simulink model "c00007M_harness"  (R2018a)
settings: Solver=FixedStepAuto  StartTime=0.0  StopTime=300  FixedStep=0.1  RelTol=1e-3
undefined symbols (not defined in the file): A1, hmax, R1, R2, sigbuilder_block, TempThreshold
(part 1 of 14)
settings Model: Creator=aarrieta  LastModifiedBy=umarkiegi

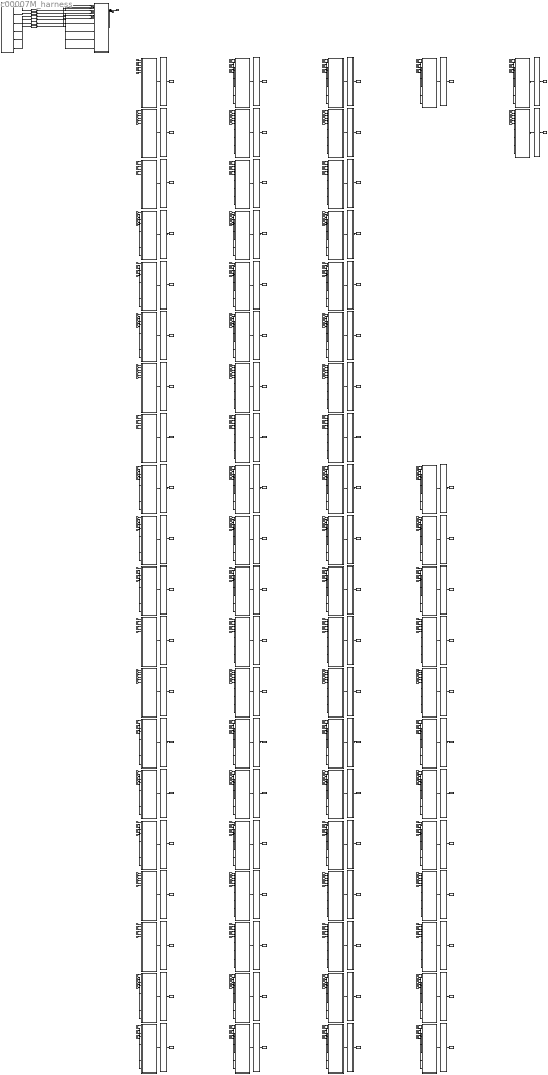
== system c00007M_harness ==
  CPSUT : Subsystem
  Eval : Subsystem
  Eval1 : Subsystem
  Eval10 : Subsystem
  Eval11 : Subsystem
  Eval12 : Subsystem
  Eval13 : Subsystem
  Eval14 : Subsystem
  Eval15 : Subsystem
  Eval16 : Subsystem
  Eval17 : Subsystem
  Eval18 : Subsystem
  Eval19 : Subsystem
  Eval2 : Subsystem
  Eval20 : Subsystem
  Eval21 : Subsystem
  Eval22 : Subsystem
  Eval23 : Subsystem
  Eval24 : Subsystem
  Eval25 : Subsystem
  Eval26 : Subsystem
  Eval27 : Subsystem
  Eval28 : Subsystem
  Eval29 : Subsystem
  Eval3 : Subsystem
  Eval30 : Subsystem
  Eval31 : Subsystem
  Eval32 : Subsystem
  Eval33 : Subsystem
  Eval34 : Subsystem
  Eval35 : Subsystem
  Eval36 : Subsystem
  Eval37 : Subsystem
  Eval38 : Subsystem
  Eval39 : Subsystem
  Eval4 : Subsystem
  Eval40 : Subsystem
  Eval41 : Subsystem
  Eval42 : Subsystem
  Eval43 : Subsystem
  Eval44 : Subsystem
  Eval45 : Subsystem
  Eval46 : Subsystem
  Eval47 : Subsystem
  Eval48 : Subsystem
  Eval49 : Subsystem
  Eval5 : Subsystem
  Eval50 : Subsystem
  Eval51 : Subsystem
  Eval52 : Subsystem
  Eval53 : Subsystem
  Eval54 : Subsystem
  Eval55 : Subsystem
  Eval56 : Subsystem
  Eval57 : Subsystem
  Eval58 : Subsystem
  Eval59 : Subsystem
  Eval6 : Subsystem
  Eval60 : Subsystem
  Eval68 : Subsystem
  Eval69 : Subsystem
  Eval7 : Subsystem
  Eval70 : Subsystem
  Eval71 : Subsystem
  Eval72 : Subsystem
  Eval73 : Subsystem
  Eval74 : Subsystem
  Eval75 : Subsystem
  Eval76 : Subsystem
  Eval77 : Subsystem
  Eval78 : Subsystem
  Eval79 : Subsystem
  Eval8 : Subsystem
  Eval80 : Subsystem
  Eval81 : Subsystem
  Eval9 : Subsystem
  Inputs : Subsystem  Tag=STV Subsys  LoadFcn=sigbuilder_block('load');  StartFcn=sigbuilder_block('start');  StopFcn=sigbuilder_block('stop');  ClipboardFcn=sigbuilder_block('clipboard');  mask(Sigbuilder block){tuvar=[0:10]}
      mask init:
      | if ~strcmp(get_param(bdroot(gcb),'SimulationStatus'),'stopped'),tuvar = sigbuilder_block('maskInit'); end
      settings: CopyFcn=sigbuilder_block('copy');  DeleteFcn=sigbuilder_block('delete');  ModelCloseFcn=sigbuilder_block('modelClose');  PreSaveFcn=sigbuilder_block('preSave');  PauseFcn=sigbuilder_block('pause');  ContinueFcn=sigbuilder_block('continue');  NameChangeFcn=sigbuilder_block('namechange');  OpenFcn=sigbuilder_block('open',[276.75 163.5 675.75 486.75 ]);  CloseFcn=sigbuilder_block('close');
      mask Display: plot(0, 0, 100, 100,[2, 2, 32, 32, 2], [68, 8, 8, 68, 68],[32, 2], [38, 38], [32, 19, 2],[53, 60, 44], [32, 17, 17, 2],[16, 16, 31, 31]);txt = getActiveGroup(gcbh);text(2, 100, txt,'verticalAlignment', 'top');
  M001 : Subsystem
  M002 : Subsystem
  M003 : Subsystem
  M004 : Subsystem
  M005 : Subsystem
  M006 : Subsystem
  M007 : Subsystem
  M008 : Subsystem
  M009 : Subsystem
  M010 : Subsystem
  M011 : Subsystem
  M012 : Subsystem
  M013 : Subsystem
  M014 : Subsystem
  M015 : Subsystem
  M016 : Subsystem
  M017 : Subsystem
  M018 : Subsystem
  M019 : Subsystem
  M020 : Subsystem
  M021 : Subsystem
  M022 : Subsystem
  M023 : Subsystem
  M024 : Subsystem
  M025 : Subsystem
  M026 : Subsystem
  M027 : Subsystem
  M028 : Subsystem
  M029 : Subsystem
  M030 : Subsystem
  M031 : Subsystem
  M032 : Subsystem
  M033 : Subsystem
  M034 : Subsystem
  M035 : Subsystem
  M036 : Subsystem
  M037 : Subsystem
  M038 : Subsystem
  M039 : Subsystem
  M040 : Subsystem
  M041 : Subsystem
  M042 : Subsystem
  M043 : Subsystem
  M044 : Subsystem
  M045 : Subsystem
  M046 : Subsystem
  M047 : Subsystem
  M048 : Subsystem
  M049 : Subsystem
  M050 : Subsystem
  M051 : Subsystem
  M052 : Subsystem
  M053 : Subsystem
  M054 : Subsystem
  M055 : Subsystem
  M056 : Subsystem
  M057 : Subsystem
  M058 : Subsystem
  M059 : Subsystem
  M060 : Subsystem
  M061 : Subsystem
  M069 : Subsystem
  M070 : Subsystem
  M071 : Subsystem
  M072 : Subsystem
  M073 : Subsystem
  M074 : Subsystem
  M075 : Subsystem
  M076 : Subsystem
  M077 : Subsystem
  M078 : Subsystem
  M079 : Subsystem
  M080 : Subsystem
  M081 : Subsystem
  M082 : Subsystem
  To Workspace : ToWorkspace  VariableName=mutant001  SampleTime=-1
  To Workspace1 : ToWorkspace  VariableName=mutant002  SampleTime=-1
  To Workspace10 : ToWorkspace  VariableName=mutant011  SampleTime=-1
  To Workspace11 : ToWorkspace  VariableName=mutant012  SampleTime=-1
  To Workspace12 : ToWorkspace  VariableName=mutant013  SampleTime=-1
  To Workspace13 : ToWorkspace  VariableName=mutant014  SampleTime=-1
  To Workspace14 : ToWorkspace  VariableName=mutant015  SampleTime=-1
  To Workspace15 : ToWorkspace  VariableName=mutant016  SampleTime=-1
  To Workspace16 : ToWorkspace  VariableName=mutant017  SampleTime=-1
  To Workspace17 : ToWorkspace  VariableName=mutant018  SampleTime=-1
  To Workspace18 : ToWorkspace  VariableName=mutant019  SampleTime=-1
  To Workspace19 : ToWorkspace  VariableName=mutant020  SampleTime=-1
  To Workspace2 : ToWorkspace  VariableName=mutant003  SampleTime=-1
  To Workspace20 : ToWorkspace  VariableName=mutant021  SampleTime=-1
  To Workspace21 : ToWorkspace  VariableName=mutant022  SampleTime=-1
  To Workspace22 : ToWorkspace  VariableName=mutant023  SampleTime=-1
  To Workspace23 : ToWorkspace  VariableName=mutant024  SampleTime=-1
  To Workspace24 : ToWorkspace  VariableName=mutant025  SampleTime=-1
  To Workspace25 : ToWorkspace  VariableName=mutant026  SampleTime=-1
  To Workspace26 : ToWorkspace  VariableName=mutant027  SampleTime=-1
  To Workspace27 : ToWorkspace  VariableName=mutant028  SampleTime=-1
  To Workspace28 : ToWorkspace  VariableName=mutant029  SampleTime=-1
  To Workspace29 : ToWorkspace  VariableName=mutant030  SampleTime=-1
  To Workspace3 : ToWorkspace  VariableName=mutant004  SampleTime=-1
  To Workspace30 : ToWorkspace  VariableName=mutant031  SampleTime=-1
  To Workspace31 : ToWorkspace  VariableName=mutant032  SampleTime=-1
  To Workspace32 : ToWorkspace  VariableName=mutant033  SampleTime=-1
  To Workspace33 : ToWorkspace  VariableName=mutant034  SampleTime=-1
  To Workspace34 : ToWorkspace  VariableName=mutant035  SampleTime=-1
  To Workspace35 : ToWorkspace  VariableName=mutant036  SampleTime=-1
  To Workspace36 : ToWorkspace  VariableName=mutant037  SampleTime=-1
  To Workspace37 : ToWorkspace  VariableName=mutant038  SampleTime=-1
  To Workspace38 : ToWorkspace  VariableName=mutant039  SampleTime=-1
  To Workspace39 : ToWorkspace  VariableName=mutant040  SampleTime=-1
  To Workspace4 : ToWorkspace  VariableName=mutant005  SampleTime=-1
  To Workspace40 : ToWorkspace  VariableName=mutant041  SampleTime=-1
  To Workspace41 : ToWorkspace  VariableName=mutant042  SampleTime=-1
  To Workspace42 : ToWorkspace  VariableName=mutant043  SampleTime=-1
  To Workspace43 : ToWorkspace  VariableName=mutant044  SampleTime=-1
  To Workspace44 : ToWorkspace  VariableName=mutant045  SampleTime=-1
  To Workspace45 : ToWorkspace  VariableName=mutant046  SampleTime=-1
  To Workspace46 : ToWorkspace  VariableName=mutant047  SampleTime=-1
  To Workspace47 : ToWorkspace  VariableName=mutant048  SampleTime=-1
  To Workspace48 : ToWorkspace  VariableName=mutant049  SampleTime=-1
  To Workspace49 : ToWorkspace  VariableName=mutant050  SampleTime=-1
  To Workspace5 : ToWorkspace  VariableName=mutant006  SampleTime=-1
  To Workspace50 : ToWorkspace  VariableName=mutant051  SampleTime=-1
  To Workspace51 : ToWorkspace  VariableName=mutant052  SampleTime=-1
  To Workspace52 : ToWorkspace  VariableName=mutant053  SampleTime=-1
  To Workspace53 : ToWorkspace  VariableName=mutant054  SampleTime=-1
  To Workspace54 : ToWorkspace  VariableName=mutant055  SampleTime=-1
  To Workspace55 : ToWorkspace  VariableName=mutant056  SampleTime=-1
  To Workspace56 : ToWorkspace  VariableName=mutant057  SampleTime=-1
  To Workspace57 : ToWorkspace  VariableName=mutant058  SampleTime=-1
  To Workspace58 : ToWorkspace  VariableName=mutant059  SampleTime=-1
  To Workspace59 : ToWorkspace  VariableName=mutant060  SampleTime=-1
  To Workspace6 : ToWorkspace  VariableName=mutant007  SampleTime=-1
  To Workspace60 : ToWorkspace  VariableName=mutant061  SampleTime=-1
  To Workspace68 : ToWorkspace  VariableName=mutant069  SampleTime=-1
  To Workspace69 : ToWorkspace  VariableName=mutant070  SampleTime=-1
  To Workspace7 : ToWorkspace  VariableName=mutant008  SampleTime=-1
  To Workspace70 : ToWorkspace  VariableName=mutant071  SampleTime=-1
  To Workspace71 : ToWorkspace  VariableName=mutant072  SampleTime=-1
  To Workspace72 : ToWorkspace  VariableName=mutant073  SampleTime=-1
  To Workspace73 : ToWorkspace  VariableName=mutant074  SampleTime=-1
  To Workspace74 : ToWorkspace  VariableName=mutant075  SampleTime=-1
  To Workspace75 : ToWorkspace  VariableName=mutant076  SampleTime=-1
  To Workspace76 : ToWorkspace  VariableName=mutant077  SampleTime=-1
  To Workspace77 : ToWorkspace  VariableName=mutant078  SampleTime=-1
  To Workspace78 : ToWorkspace  VariableName=mutant079  SampleTime=-1
  To Workspace79 : ToWorkspace  VariableName=mutant080  SampleTime=-1
  To Workspace8 : ToWorkspace  VariableName=mutant009  SampleTime=-1
  To Workspace80 : ToWorkspace  VariableName=mutant081  SampleTime=-1
  To Workspace81 : ToWorkspace  VariableName=mutant082  SampleTime=-1
  To Workspace9 : ToWorkspace  VariableName=mutant010  SampleTime=-1
  dtc_CT1 : DataTypeConversion
  dtc_E1 : DataTypeConversion
  dtc_EB1 : DataTypeConversion
  dtc_F1 : DataTypeConversion
  dtc_MR1 : DataTypeConversion
  dtc_T1 : DataTypeConversion
  LL1 : Outport
  tag scope: out1=global
  wires:
  CPSUT/1(LL1) -> [out1], LL1/1
  [in1] -> M001/1(CT1)
  [in2] -> M001/2(F1)
  [in3] -> M001/3(E1)
  [in4] -> M001/4(MR1)
  [in5] -> M001/5(T1)
  [in6] -> M001/6(EB1)
  Eval/1(Out1) -> To Workspace/1
  M001/1(LL1) -> Eval/1(In1)
  [in1] -> M002/1(CT1)
  [in2] -> M002/2(F1)
  [in3] -> M002/3(E1)
  [in4] -> M002/4(MR1)
  [in5] -> M002/5(T1)
  [in6] -> M002/6(EB1)
  M002/1(LL1) -> Eval1/1(In1)
  Eval1/1(Out1) -> To Workspace1/1
  [in1] -> M003/1(CT1)
  [in2] -> M003/2(F1)
  [in3] -> M003/3(E1)
  [in4] -> M003/4(MR1)
  [in5] -> M003/5(T1)
  [in6] -> M003/6(EB1)
  M003/1(LL1) -> Eval2/1(In1)
  Eval2/1(Out1) -> To Workspace2/1
  [in1] -> M004/1(CT1)
  [in2] -> M004/2(F1)
  [in3] -> M004/3(E1)
  [in4] -> M004/4(MR1)
  [in5] -> M004/5(T1)
  [in6] -> M004/6(EB1)
  M004/1(LL1) -> Eval3/1(In1)
  Eval3/1(Out1) -> To Workspace3/1
  [in1] -> M005/1(CT1)
  [in2] -> M005/2(F1)
  [in3] -> M005/3(E1)
  [in4] -> M005/4(MR1)
  [in5] -> M005/5(T1)
  [in6] -> M005/6(EB1)
  M005/1(LL1) -> Eval4/1(In1)
  Eval4/1(Out1) -> To Workspace4/1
  [in1] -> M006/1(CT1)
  [in2] -> M006/2(F1)
  [in3] -> M006/3(E1)
  [in4] -> M006/4(MR1)
  [in5] -> M006/5(T1)
  [in6] -> M006/6(EB1)
  M006/1(LL1) -> Eval5/1(In1)
  Eval5/1(Out1) -> To Workspace5/1
  [in1] -> M007/1(CT1)
  [in2] -> M007/2(F1)
  [in3] -> M007/3(E1)
  [in4] -> M007/4(MR1)
  [in5] -> M007/5(T1)
  [in6] -> M007/6(EB1)
  M007/1(LL1) -> Eval6/1(In1)
  Eval6/1(Out1) -> To Workspace6/1
  [in1] -> M008/1(CT1)
  [in2] -> M008/2(F1)
  [in3] -> M008/3(E1)
  [in4] -> M008/4(MR1)
  [in5] -> M008/5(T1)
  [in6] -> M008/6(EB1)
  M008/1(LL1) -> Eval7/1(In1)
  Eval7/1(Out1) -> To Workspace7/1
  [in1] -> M009/1(CT1)
  [in2] -> M009/2(F1)
  [in3] -> M009/3(E1)
  [in4] -> M009/4(MR1)
  [in5] -> M009/5(T1)
  [in6] -> M009/6(EB1)
  M009/1(LL1) -> Eval8/1(In1)
  Eval8/1(Out1) -> To Workspace8/1
  [in1] -> M010/1(CT1)
  [in2] -> M010/2(F1)
  [in3] -> M010/3(E1)
  [in4] -> M010/4(MR1)
  [in5] -> M010/5(T1)
  [in6] -> M010/6(EB1)
  M010/1(LL1) -> Eval9/1(In1)
  Eval9/1(Out1) -> To Workspace9/1
  [in1] -> M011/1(CT1)
  [in2] -> M011/2(F1)
  [in3] -> M011/3(E1)
  [in4] -> M011/4(MR1)
  [in5] -> M011/5(T1)
  [in6] -> M011/6(EB1)
  M011/1(LL1) -> Eval10/1(In1)
  Eval10/1(Out1) -> To Workspace10/1
  [in1] -> M012/1(CT1)
  [in2] -> M012/2(F1)
  [in3] -> M012/3(E1)
  [in4] -> M012/4(MR1)
  [in5] -> M012/5(T1)
  [in6] -> M012/6(EB1)
  M012/1(LL1) -> Eval11/1(In1)
  Eval11/1(Out1) -> To Workspace11/1
  [in1] -> M013/1(CT1)
  [in2] -> M013/2(F1)
  [in3] -> M013/3(E1)
  [in4] -> M013/4(MR1)
  [in5] -> M013/5(T1)
  [in6] -> M013/6(EB1)
  M013/1(LL1) -> Eval12/1(In1)
  Eval12/1(Out1) -> To Workspace12/1
  [in1] -> M014/1(CT1)
  [in2] -> M014/2(F1)
  [in3] -> M014/3(E1)
  [in4] -> M014/4(MR1)
  [in5] -> M014/5(T1)
  [in6] -> M014/6(EB1)
  M014/1(LL1) -> Eval13/1(In1)
  Eval13/1(Out1) -> To Workspace13/1
  [in1] -> M015/1(CT1)
  [in2] -> M015/2(F1)
  [in3] -> M015/3(E1)
  [in4] -> M015/4(MR1)
  [in5] -> M015/5(T1)
  [in6] -> M015/6(EB1)
  M015/1(LL1) -> Eval14/1(In1)
  Eval14/1(Out1) -> To Workspace14/1
  [in1] -> M016/1(CT1)
  [in2] -> M016/2(F1)
  [in3] -> M016/3(E1)
  [in4] -> M016/4(MR1)
  [in5] -> M016/5(T1)
  [in6] -> M016/6(EB1)
  M016/1(LL1) -> Eval15/1(In1)
  Eval15/1(Out1) -> To Workspace15/1
  [in1] -> M017/1(CT1)
  [in2] -> M017/2(F1)
  [in3] -> M017/3(E1)
  [in4] -> M017/4(MR1)
  [in5] -> M017/5(T1)
  [in6] -> M017/6(EB1)
  M017/1(LL1) -> Eval16/1(In1)
  Eval16/1(Out1) -> To Workspace16/1
  [in1] -> M018/1(CT1)
  [in2] -> M018/2(F1)
  [in3] -> M018/3(E1)
  [in4] -> M018/4(MR1)
  [in5] -> M018/5(T1)
  [in6] -> M018/6(EB1)
  M018/1(LL1) -> Eval17/1(In1)
  Eval17/1(Out1) -> To Workspace17/1
  [in1] -> M019/1(CT1)
  [in2] -> M019/2(F1)
  [in3] -> M019/3(E1)
  [in4] -> M019/4(MR1)
  [in5] -> M019/5(T1)
  [in6] -> M019/6(EB1)
  M019/1(LL1) -> Eval18/1(In1)
  Eval18/1(Out1) -> To Workspace18/1
  [in1] -> M020/1(CT1)
  [in2] -> M020/2(F1)
  [in3] -> M020/3(E1)
  [in4] -> M020/4(MR1)
  [in5] -> M020/5(T1)
  [in6] -> M020/6(EB1)
  M020/1(LL1) -> Eval19/1(In1)
  Eval19/1(Out1) -> To Workspace19/1
  [in1] -> M021/1(CT1)
  [in2] -> M021/2(F1)
  [in3] -> M021/3(E1)
  [in4] -> M021/4(MR1)
  [in5] -> M021/5(T1)
  [in6] -> M021/6(EB1)
  M021/1(LL1) -> Eval20/1(In1)
  Eval20/1(Out1) -> To Workspace20/1
  [in1] -> M022/1(CT1)
  [in2] -> M022/2(F1)
  [in3] -> M022/3(E1)
  [in4] -> M022/4(MR1)
  [in5] -> M022/5(T1)
  [in6] -> M022/6(EB1)
  M022/1(LL1) -> Eval21/1(In1)
  Eval21/1(Out1) -> To Workspace21/1
  [in1] -> M023/1(CT1)
  [in2] -> M023/2(F1)
  [in3] -> M023/3(E1)
  [in4] -> M023/4(MR1)
  [in5] -> M023/5(T1)
  [in6] -> M023/6(EB1)
  M023/1(LL1) -> Eval22/1(In1)
  Eval22/1(Out1) -> To Workspace22/1
  [in1] -> M024/1(CT1)
  [in2] -> M024/2(F1)
  [in3] -> M024/3(E1)
  [in4] -> M024/4(MR1)
  [in5] -> M024/5(T1)
  [in6] -> M024/6(EB1)
  M024/1(LL1) -> Eval23/1(In1)
  Eval23/1(Out1) -> To Workspace23/1
  [in1] -> M025/1(CT1)
  [in2] -> M025/2(F1)
  [in3] -> M025/3(E1)
  [in4] -> M025/4(MR1)
  [in5] -> M025/5(T1)
  [in6] -> M025/6(EB1)
  M025/1(LL1) -> Eval24/1(In1)
  Eval24/1(Out1) -> To Workspace24/1
  [in1] -> M026/1(CT1)
  [in2] -> M026/2(F1)
  [in3] -> M026/3(E1)
  [in4] -> M026/4(MR1)
  [in5] -> M026/5(T1)
  [in6] -> M026/6(EB1)
  M026/1(LL1) -> Eval25/1(In1)
  Eval25/1(Out1) -> To Workspace25/1
  [in1] -> M027/1(CT1)
  [in2] -> M027/2(F1)
  [in3] -> M027/3(E1)
  [in4] -> M027/4(MR1)
  [in5] -> M027/5(T1)
  [in6] -> M027/6(EB1)
  M027/1(LL1) -> Eval26/1(In1)
  Eval26/1(Out1) -> To Workspace26/1
  [in1] -> M028/1(CT1)
  [in2] -> M028/2(F1)
  [in3] -> M028/3(E1)
  [in4] -> M028/4(MR1)
  [in5] -> M028/5(T1)
  [in6] -> M028/6(EB1)
  M028/1(LL1) -> Eval27/1(In1)
  Eval27/1(Out1) -> To Workspace27/1
  [in1] -> M029/1(CT1)
  [in2] -> M029/2(F1)
  [in3] -> M029/3(E1)
  [in4] -> M029/4(MR1)
  [in5] -> M029/5(T1)
  [in6] -> M029/6(EB1)
  M029/1(LL1) -> Eval28/1(In1)
  Eval28/1(Out1) -> To Workspace28/1
  [in1] -> M030/1(CT1)
  [in2] -> M030/2(F1)
  [in3] -> M030/3(E1)
  [in4] -> M030/4(MR1)
  [in5] -> M030/5(T1)
  [in6] -> M030/6(EB1)
  M030/1(LL1) -> Eval29/1(In1)
  Eval29/1(Out1) -> To Workspace29/1
  [in1] -> M031/1(CT1)
  [in2] -> M031/2(F1)
  [in3] -> M031/3(E1)
  [in4] -> M031/4(MR1)
  [in5] -> M031/5(T1)
  [in6] -> M031/6(EB1)
  M031/1(LL1) -> Eval30/1(In1)
  Eval30/1(Out1) -> To Workspace30/1
  [in1] -> M032/1(CT1)
  [in2] -> M032/2(F1)
  [in3] -> M032/3(E1)
  [in4] -> M032/4(MR1)
  [in5] -> M032/5(T1)
  [in6] -> M032/6(EB1)
  M032/1(LL1) -> Eval31/1(In1)
  Eval31/1(Out1) -> To Workspace31/1
  [in1] -> M033/1(CT1)
  [in2] -> M033/2(F1)
  [in3] -> M033/3(E1)
  [in4] -> M033/4(MR1)
  [in5] -> M033/5(T1)
  [in6] -> M033/6(EB1)
  M033/1(LL1) -> Eval32/1(In1)
  Eval32/1(Out1) -> To Workspace32/1
  [in1] -> M034/1(CT1)
  [in2] -> M034/2(F1)
  [in3] -> M034/3(E1)
  [in4] -> M034/4(MR1)
  [in5] -> M034/5(T1)
  [in6] -> M034/6(EB1)
  M034/1(LL1) -> Eval33/1(In1)
  Eval33/1(Out1) -> To Workspace33/1
  [in1] -> M035/1(CT1)
  [in2] -> M035/2(F1)
  [in3] -> M035/3(E1)
  [in4] -> M035/4(MR1)
  [in5] -> M035/5(T1)
  [in6] -> M035/6(EB1)
  M035/1(LL1) -> Eval34/1(In1)
  Eval34/1(Out1) -> To Workspace34/1
  [in1] -> M036/1(CT1)
  [in2] -> M036/2(F1)
  [in3] -> M036/3(E1)
  [in4] -> M036/4(MR1)
  [in5] -> M036/5(T1)
  [in6] -> M036/6(EB1)
  M036/1(LL1) -> Eval35/1(In1)
  Eval35/1(Out1) -> To Workspace35/1
  [in1] -> M037/1(CT1)
  [in2] -> M037/2(F1)
  [in3] -> M037/3(E1)
  [in4] -> M037/4(MR1)
  [in5] -> M037/5(T1)
  [in6] -> M037/6(EB1)
  M037/1(LL1) -> Eval36/1(In1)
  Eval36/1(Out1) -> To Workspace36/1
  [in1] -> M038/1(CT1)
  [in2] -> M038/2(F1)
  [in3] -> M038/3(E1)
  [in4] -> M038/4(MR1)
  [in5] -> M038/5(T1)
  [in6] -> M038/6(EB1)
  M038/1(LL1) -> Eval37/1(In1)
  Eval37/1(Out1) -> To Workspace37/1
  [in1] -> M039/1(CT1)
  [in2] -> M039/2(F1)
  [in3] -> M039/3(E1)
  [in4] -> M039/4(MR1)
  [in5] -> M039/5(T1)
  [in6] -> M039/6(EB1)
  M039/1(LL1) -> Eval38/1(In1)
  Eval38/1(Out1) -> To Workspace38/1
  [in1] -> M040/1(CT1)
  [in2] -> M040/2(F1)
  [in3] -> M040/3(E1)
  [in4] -> M040/4(MR1)
  [in5] -> M040/5(T1)
  [in6] -> M040/6(EB1)
  M040/1(LL1) -> Eval39/1(In1)
  Eval39/1(Out1) -> To Workspace39/1
  [in1] -> M041/1(CT1)
  [in2] -> M041/2(F1)
  [in3] -> M041/3(E1)
  [in4] -> M041/4(MR1)
  [in5] -> M041/5(T1)
  [in6] -> M041/6(EB1)
  M041/1(LL1) -> Eval40/1(In1)
  Eval40/1(Out1) -> To Workspace40/1
  [in1] -> M042/1(CT1)
  [in2] -> M042/2(F1)
  [in3] -> M042/3(E1)
  [in4] -> M042/4(MR1)
  [in5] -> M042/5(T1)
  [in6] -> M042/6(EB1)
  M042/1(LL1) -> Eval41/1(In1)
  Eval41/1(Out1) -> To Workspace41/1
  [in1] -> M043/1(CT1)
  [in2] -> M043/2(F1)
  [in3] -> M043/3(E1)
  [in4] -> M043/4(MR1)
  [in5] -> M043/5(T1)
  [in6] -> M043/6(EB1)
  M043/1(LL1) -> Eval42/1(In1)
  Eval42/1(Out1) -> To Workspace42/1
  [in1] -> M044/1(CT1)
  [in2] -> M044/2(F1)
  [in3] -> M044/3(E1)
  [in4] -> M044/4(MR1)
  [in5] -> M044/5(T1)
  [in6] -> M044/6(EB1)
  M044/1(LL1) -> Eval43/1(In1)
  Eval43/1(Out1) -> To Workspace43/1
  [in1] -> M045/1(CT1)
  [in2] -> M045/2(F1)
  [in3] -> M045/3(E1)
  [in4] -> M045/4(MR1)
  [in5] -> M045/5(T1)
  [in6] -> M045/6(EB1)
  M045/1(LL1) -> Eval44/1(In1)
  Eval44/1(Out1) -> To Workspace44/1
  [in1] -> M046/1(CT1)
  [in2] -> M046/2(F1)
  [in3] -> M046/3(E1)
  [in4] -> M046/4(MR1)
  [in5] -> M046/5(T1)
  [in6] -> M046/6(EB1)
  M046/1(LL1) -> Eval45/1(In1)
  Eval45/1(Out1) -> To Workspace45/1
  [in1] -> M047/1(CT1)
  [in2] -> M047/2(F1)
  [in3] -> M047/3(E1)
  [in4] -> M047/4(MR1)
  [in5] -> M047/5(T1)
  [in6] -> M047/6(EB1)
  M047/1(LL1) -> Eval46/1(In1)
  Eval46/1(Out1) -> To Workspace46/1
  [in1] -> M048/1(CT1)
  [in2] -> M048/2(F1)
  [in3] -> M048/3(E1)
  [in4] -> M048/4(MR1)
  [in5] -> M048/5(T1)
  [in6] -> M048/6(EB1)
  M048/1(LL1) -> Eval47/1(In1)
  Eval47/1(Out1) -> To Workspace47/1
  [in1] -> M049/1(CT1)
  [in2] -> M049/2(F1)
  [in3] -> M049/3(E1)
  [in4] -> M049/4(MR1)
  [in5] -> M049/5(T1)
  [in6] -> M049/6(EB1)
  M049/1(LL1) -> Eval48/1(In1)
  Eval48/1(Out1) -> To Workspace48/1
  [in1] -> M050/1(CT1)
  [in2] -> M050/2(F1)
  [in3] -> M050/3(E1)
  [in4] -> M050/4(MR1)
  [in5] -> M050/5(T1)
  [in6] -> M050/6(EB1)
  M050/1(LL1) -> Eval49/1(In1)
  Eval49/1(Out1) -> To Workspace49/1
  [in1] -> M051/1(CT1)
  [in2] -> M051/2(F1)
  [in3] -> M051/3(E1)
  [in4] -> M051/4(MR1)
  [in5] -> M051/5(T1)
  [in6] -> M051/6(EB1)
  M051/1(LL1) -> Eval50/1(In1)
  Eval50/1(Out1) -> To Workspace50/1
  [in1] -> M052/1(CT1)
  [in2] -> M052/2(F1)
  [in3] -> M052/3(E1)
  [in4] -> M052/4(MR1)
  [in5] -> M052/5(T1)
  [in6] -> M052/6(EB1)
  M052/1(LL1) -> Eval51/1(In1)
  Eval51/1(Out1) -> To Workspace51/1
  [in1] -> M053/1(CT1)
  [in2] -> M053/2(F1)
  [in3] -> M053/3(E1)
  [in4] -> M053/4(MR1)
  [in5] -> M053/5(T1)
  [in6] -> M053/6(EB1)
  M053/1(LL1) -> Eval52/1(In1)
  Eval52/1(Out1) -> To Workspace52/1
  [in1] -> M054/1(CT1)
  [in2] -> M054/2(F1)
  [in3] -> M054/3(E1)
  [in4] -> M054/4(MR1)
  [in5] -> M054/5(T1)
  [in6] -> M054/6(EB1)
  M054/1(LL1) -> Eval53/1(In1)
  Eval53/1(Out1) -> To Workspace53/1
  [in1] -> M055/1(CT1)
  [in2] -> M055/2(F1)
  [in3] -> M055/3(E1)
  [in4] -> M055/4(MR1)
  [in5] -> M055/5(T1)
  [in6] -> M055/6(EB1)
  M055/1(LL1) -> Eval54/1(In1)
  Eval54/1(Out1) -> To Workspace54/1
  [in1] -> M056/1(CT1)
  [in2] -> M056/2(F1)
  [in3] -> M056/3(E1)
  [in4] -> M056/4(MR1)
  [in5] -> M056/5(T1)
  [in6] -> M056/6(EB1)
  M056/1(LL1) -> Eval55/1(In1)
  Eval55/1(Out1) -> To Workspace55/1
  [in1] -> M057/1(CT1)
  [in2] -> M057/2(F1)
  [in3] -> M057/3(E1)
  [in4] -> M057/4(MR1)
  [in5] -> M057/5(T1)
  [in6] -> M057/6(EB1)
  M057/1(LL1) -> Eval56/1(In1)
  Eval56/1(Out1) -> To Workspace56/1
  [in1] -> M058/1(CT1)
  [in2] -> M058/2(F1)
  [in3] -> M058/3(E1)
  [in4] -> M058/4(MR1)
  [in5] -> M058/5(T1)
  [in6] -> M058/6(EB1)
  M058/1(LL1) -> Eval57/1(In1)
  Eval57/1(Out1) -> To Workspace57/1
  [in1] -> M059/1(CT1)
  [in2] -> M059/2(F1)
  [in3] -> M059/3(E1)
  [in4] -> M059/4(MR1)
  [in5] -> M059/5(T1)
  [in6] -> M059/6(EB1)
  M059/1(LL1) -> Eval58/1(In1)
  Eval58/1(Out1) -> To Workspace58/1
  [in1] -> M060/1(CT1)
  [in2] -> M060/2(F1)
  [in3] -> M060/3(E1)
  [in4] -> M060/4(MR1)
  [in5] -> M060/5(T1)
  [in6] -> M060/6(EB1)
  M060/1(LL1) -> Eval59/1(In1)
  Eval59/1(Out1) -> To Workspace59/1
  [in1] -> M061/1(CT1)
  [in2] -> M061/2(F1)
  [in3] -> M061/3(E1)
  [in4] -> M061/4(MR1)
  [in5] -> M061/5(T1)
  [in6] -> M061/6(EB1)
  M061/1(LL1) -> Eval60/1(In1)
  Eval60/1(Out1) -> To Workspace60/1
  [in1] -> M069/1(CT1)
  [in2] -> M069/2(F1)
  [in3] -> M069/3(E1)
  [in4] -> M069/4(MR1)
  [in5] -> M069/5(T1)
  [in6] -> M069/6(EB1)
  M069/1(LL1) -> Eval68/1(In1)
  Eval68/1(Out1) -> To Workspace68/1
  [in1] -> M070/1(CT1)
  [in2] -> M070/2(F1)
  [in3] -> M070/3(E1)
  [in4] -> M070/4(MR1)
  [in5] -> M070/5(T1)
  [in6] -> M070/6(EB1)
  M070/1(LL1) -> Eval69/1(In1)
  Eval69/1(Out1) -> To Workspace69/1
  [in1] -> M071/1(CT1)
  [in2] -> M071/2(F1)
  [in3] -> M071/3(E1)
  [in4] -> M071/4(MR1)
  [in5] -> M071/5(T1)
  [in6] -> M071/6(EB1)
  M071/1(LL1) -> Eval70/1(In1)
  Eval70/1(Out1) -> To Workspace70/1
  [in1] -> M072/1(CT1)
  [in2] -> M072/2(F1)
  [in3] -> M072/3(E1)
  [in4] -> M072/4(MR1)
  [in5] -> M072/5(T1)
  [in6] -> M072/6(EB1)
  M072/1(LL1) -> Eval71/1(In1)
  Eval71/1(Out1) -> To Workspace71/1
  [in1] -> M073/1(CT1)
  [in2] -> M073/2(F1)
  [in3] -> M073/3(E1)
  [in4] -> M073/4(MR1)
  [in5] -> M073/5(T1)
  [in6] -> M073/6(EB1)
  M073/1(LL1) -> Eval72/1(In1)
  Eval72/1(Out1) -> To Workspace72/1
  [in1] -> M074/1(CT1)
  [in2] -> M074/2(F1)
  [in3] -> M074/3(E1)
  [in4] -> M074/4(MR1)
  [in5] -> M074/5(T1)
  [in6] -> M074/6(EB1)
  M074/1(LL1) -> Eval73/1(In1)
  Eval73/1(Out1) -> To Workspace73/1
  [in1] -> M075/1(CT1)
  [in2] -> M075/2(F1)
  [in3] -> M075/3(E1)
  [in4] -> M075/4(MR1)
  [in5] -> M075/5(T1)
  [in6] -> M075/6(EB1)
  M075/1(LL1) -> Eval74/1(In1)
  Eval74/1(Out1) -> To Workspace74/1
  [in1] -> M076/1(CT1)
  [in2] -> M076/2(F1)
  [in3] -> M076/3(E1)
  [in4] -> M076/4(MR1)
  [in5] -> M076/5(T1)
  [in6] -> M076/6(EB1)
  M076/1(LL1) -> Eval75/1(In1)
  Eval75/1(Out1) -> To Workspace75/1
  [in1] -> M077/1(CT1)
  [in2] -> M077/2(F1)
  [in3] -> M077/3(E1)
  [in4] -> M077/4(MR1)
  [in5] -> M077/5(T1)
  [in6] -> M077/6(EB1)
  M077/1(LL1) -> Eval76/1(In1)
  Eval76/1(Out1) -> To Workspace76/1
  [in1] -> M078/1(CT1)
  [in2] -> M078/2(F1)
  [in3] -> M078/3(E1)
  [in4] -> M078/4(MR1)
  [in5] -> M078/5(T1)
  [in6] -> M078/6(EB1)
  M078/1(LL1) -> Eval77/1(In1)
  Eval77/1(Out1) -> To Workspace77/1
  [in1] -> M079/1(CT1)
  [in2] -> M079/2(F1)
  [in3] -> M079/3(E1)
  [in4] -> M079/4(MR1)
  [in5] -> M079/5(T1)
  [in6] -> M079/6(EB1)
  M079/1(LL1) -> Eval78/1(In1)
  Eval78/1(Out1) -> To Workspace78/1
  [in1] -> M080/1(CT1)
  [in2] -> M080/2(F1)
  [in3] -> M080/3(E1)
  [in4] -> M080/4(MR1)
  [in5] -> M080/5(T1)
  [in6] -> M080/6(EB1)
  M080/1(LL1) -> Eval79/1(In1)
  Eval79/1(Out1) -> To Workspace79/1
  [in1] -> M081/1(CT1)
  [in2] -> M081/2(F1)
  [in3] -> M081/3(E1)
  [in4] -> M081/4(MR1)
  [in5] -> M081/5(T1)
  [in6] -> M081/6(EB1)
  M081/1(LL1) -> Eval80/1(In1)
  Eval80/1(Out1) -> To Workspace80/1
  [in1] -> M082/1(CT1)
  [in2] -> M082/2(F1)
  [in3] -> M082/3(E1)
  [in4] -> M082/4(MR1)
  [in5] -> M082/5(T1)
  [in6] -> M082/6(EB1)
  M082/1(LL1) -> Eval81/1(In1)
  Eval81/1(Out1) -> To Workspace81/1
  Inputs/1(CT1) -> dtc_CT1/1
  dtc_CT1/1 -> CPSUT/1(CT1), [in1]
  Inputs/2(F1) -> dtc_F1/1
  dtc_F1/1 -> CPSUT/2(F1), [in2]
  Inputs/3(E1) -> dtc_E1/1
  dtc_E1/1 -> CPSUT/3(E1), [in3]
  Inputs/4(MR1) -> dtc_MR1/1
  dtc_MR1/1 -> CPSUT/4(MR1), [in4]
  Inputs/5(T1) -> dtc_T1/1
  dtc_T1/1 -> CPSUT/5(T1), [in5]
  Inputs/6(EB1) -> dtc_EB1/1
  dtc_EB1/1 -> CPSUT/6(EB1), [in6]

== system c00007M_harness/CPSUT ==
  note: VALUES
      | ---------------------------------
      | ControlType = 1 | 2 | 3
      | FillTank = 0 | 1
      | EmptyTank = 0 | 1
      | ManualReference between 0 and 1
      | Tempreature between 0 and 100
      | EmergencyButton = 0 | 1
      | LiquidLevel between 0 and 1 (hmax)
  note: Inputs For Tank2
  note: NAMES
      | --------------------------------------------
      | CT1 = ControlType Tank 1
      | F1 = Fill Tank 1
      | E1 = Empty Tank 1
      | MR1 = Manual Reference Tank1
      | T1 = Temperature Tank 1
      | EB1 = Emergency Button Tank 1
      | LL1 = Liquid Level 1
  note: Inputs For Tank3
  note: Inputs For Tank1
  CT1 : Inport
  F1 : Inport  Port=2
  E1 : Inport  Port=3
  MR1 : Inport  Port=4
  T1 : Inport  Port=5
  EB1 : Inport  Port=6
  Tank1 : Subsystem
  LL1 : Outport
  wires:
  EB1/1 -> Tank1/6(EB1)
  MR1/1 -> Tank1/4(MR1)
  T1/1 -> Tank1/5(T1)
  Tank1/1(LL1) -> LL1/1
  F1/1 -> Tank1/2(F1)
  E1/1 -> Tank1/3(E1)
  CT1/1 -> Tank1/1(CT1)

== system c00007M_harness/Eval ==
  In1 : Inport
  Constant2 : Constant
  Constant3 : Constant
  Data Type Conversion : DataTypeConversion
  Memory1 : Memory  InitialCondition=1
  MinMax : MinMax  Inputs=3
  MinMax1 : MinMax  Inputs=2
  ROOut1 : RelationalOperator  Operator===  OutDataTypeStr=boolean  RndMeth=Simplest
  Out1 : Outport
  wires:
  MinMax/1 -> Out1/1
  [out1] -> ROOut1/2
  In1/1 -> ROOut1/1
  Memory1/1 -> MinMax1/2
  ROOut1/1 -> Data Type Conversion/1
  MinMax1/1 -> MinMax/1, Memory1/1
  Data Type Conversion/1 -> MinMax1/1
  Constant2/1 -> MinMax/2
  Constant3/1 -> MinMax/3

== system c00007M_harness/Eval1 ==
  In1 : Inport
  Constant2 : Constant
  Constant3 : Constant
  Data Type Conversion : DataTypeConversion
  Memory1 : Memory  InitialCondition=1
  MinMax : MinMax  Inputs=3
  MinMax1 : MinMax  Inputs=2
  ROOut1 : RelationalOperator  Operator===  OutDataTypeStr=boolean  RndMeth=Simplest
  Out1 : Outport
  wires:
  Data Type Conversion/1 -> MinMax1/1
  MinMax1/1 -> Memory1/1, MinMax/1
  ROOut1/1 -> Data Type Conversion/1
  Memory1/1 -> MinMax1/2
  In1/1 -> ROOut1/1
  [out1] -> ROOut1/2
  MinMax/1 -> Out1/1
  Constant2/1 -> MinMax/2
  Constant3/1 -> MinMax/3

== system c00007M_harness/Eval10 ==
  In1 : Inport
  Constant2 : Constant
  Constant3 : Constant
  Data Type Conversion : DataTypeConversion
  Memory1 : Memory  InitialCondition=1
  MinMax : MinMax  Inputs=3
  MinMax1 : MinMax  Inputs=2
  ROOut1 : RelationalOperator  Operator===  OutDataTypeStr=boolean  RndMeth=Simplest
  Out1 : Outport
  wires:
  Data Type Conversion/1 -> MinMax1/1
  MinMax1/1 -> Memory1/1, MinMax/1
  ROOut1/1 -> Data Type Conversion/1
  Memory1/1 -> MinMax1/2
  In1/1 -> ROOut1/1
  [out1] -> ROOut1/2
  MinMax/1 -> Out1/1
  Constant2/1 -> MinMax/2
  Constant3/1 -> MinMax/3

== system c00007M_harness/Eval11 ==
  In1 : Inport
  Constant2 : Constant
  Constant3 : Constant
  Data Type Conversion : DataTypeConversion
  Memory1 : Memory  InitialCondition=1
  MinMax : MinMax  Inputs=3
  MinMax1 : MinMax  Inputs=2
  ROOut1 : RelationalOperator  Operator===  OutDataTypeStr=boolean  RndMeth=Simplest
  Out1 : Outport
  wires:
  Data Type Conversion/1 -> MinMax1/1
  MinMax1/1 -> Memory1/1, MinMax/1
  ROOut1/1 -> Data Type Conversion/1
  Memory1/1 -> MinMax1/2
  In1/1 -> ROOut1/1
  [out1] -> ROOut1/2
  MinMax/1 -> Out1/1
  Constant2/1 -> MinMax/2
  Constant3/1 -> MinMax/3

== system c00007M_harness/Eval12 ==
  In1 : Inport
  Constant2 : Constant
  Constant3 : Constant
  Data Type Conversion : DataTypeConversion
  Memory1 : Memory  InitialCondition=1
  MinMax : MinMax  Inputs=3
  MinMax1 : MinMax  Inputs=2
  ROOut1 : RelationalOperator  Operator===  OutDataTypeStr=boolean  RndMeth=Simplest
  Out1 : Outport
  wires:
  Data Type Conversion/1 -> MinMax1/1
  MinMax1/1 -> Memory1/1, MinMax/1
  ROOut1/1 -> Data Type Conversion/1
  Memory1/1 -> MinMax1/2
  In1/1 -> ROOut1/1
  [out1] -> ROOut1/2
  MinMax/1 -> Out1/1
  Constant2/1 -> MinMax/2
  Constant3/1 -> MinMax/3

== system c00007M_harness/Eval13 ==
  In1 : Inport
  Constant2 : Constant
  Constant3 : Constant
  Data Type Conversion : DataTypeConversion
  Memory1 : Memory  InitialCondition=1
  MinMax : MinMax  Inputs=3
  MinMax1 : MinMax  Inputs=2
  ROOut1 : RelationalOperator  Operator===  OutDataTypeStr=boolean  RndMeth=Simplest
  Out1 : Outport
  wires:
  Data Type Conversion/1 -> MinMax1/1
  MinMax1/1 -> Memory1/1, MinMax/1
  ROOut1/1 -> Data Type Conversion/1
  Memory1/1 -> MinMax1/2
  In1/1 -> ROOut1/1
  [out1] -> ROOut1/2
  MinMax/1 -> Out1/1
  Constant2/1 -> MinMax/2
  Constant3/1 -> MinMax/3

== system c00007M_harness/Eval14 ==
  In1 : Inport
  Constant2 : Constant
  Constant3 : Constant
  Data Type Conversion : DataTypeConversion
  Memory1 : Memory  InitialCondition=1
  MinMax : MinMax  Inputs=3
  MinMax1 : MinMax  Inputs=2
  ROOut1 : RelationalOperator  Operator===  OutDataTypeStr=boolean  RndMeth=Simplest
  Out1 : Outport
  wires:
  Data Type Conversion/1 -> MinMax1/1
  MinMax1/1 -> Memory1/1, MinMax/1
  ROOut1/1 -> Data Type Conversion/1
  Memory1/1 -> MinMax1/2
  In1/1 -> ROOut1/1
  [out1] -> ROOut1/2
  MinMax/1 -> Out1/1
  Constant2/1 -> MinMax/2
  Constant3/1 -> MinMax/3

== system c00007M_harness/Eval15 ==
  In1 : Inport
  Constant2 : Constant
  Constant3 : Constant
  Data Type Conversion : DataTypeConversion
  Memory1 : Memory  InitialCondition=1
  MinMax : MinMax  Inputs=3
  MinMax1 : MinMax  Inputs=2
  ROOut1 : RelationalOperator  Operator===  OutDataTypeStr=boolean  RndMeth=Simplest
  Out1 : Outport
  wires:
  Data Type Conversion/1 -> MinMax1/1
  MinMax1/1 -> Memory1/1, MinMax/1
  ROOut1/1 -> Data Type Conversion/1
  Memory1/1 -> MinMax1/2
  In1/1 -> ROOut1/1
  [out1] -> ROOut1/2
  MinMax/1 -> Out1/1
  Constant2/1 -> MinMax/2
  Constant3/1 -> MinMax/3

== system c00007M_harness/Eval16 ==
  In1 : Inport
  Constant2 : Constant
  Constant3 : Constant
  Data Type Conversion : DataTypeConversion
  Memory1 : Memory  InitialCondition=1
  MinMax : MinMax  Inputs=3
  MinMax1 : MinMax  Inputs=2
  ROOut1 : RelationalOperator  Operator===  OutDataTypeStr=boolean  RndMeth=Simplest
  Out1 : Outport
  wires:
  Data Type Conversion/1 -> MinMax1/1
  MinMax1/1 -> Memory1/1, MinMax/1
  ROOut1/1 -> Data Type Conversion/1
  Memory1/1 -> MinMax1/2
  In1/1 -> ROOut1/1
  [out1] -> ROOut1/2
  MinMax/1 -> Out1/1
  Constant2/1 -> MinMax/2
  Constant3/1 -> MinMax/3

== system c00007M_harness/Eval17 ==
  In1 : Inport
  Constant2 : Constant
  Constant3 : Constant
  Data Type Conversion : DataTypeConversion
  Memory1 : Memory  InitialCondition=1
  MinMax : MinMax  Inputs=3
  MinMax1 : MinMax  Inputs=2
  ROOut1 : RelationalOperator  Operator===  OutDataTypeStr=boolean  RndMeth=Simplest
  Out1 : Outport
  wires:
  Data Type Conversion/1 -> MinMax1/1
  MinMax1/1 -> Memory1/1, MinMax/1
  ROOut1/1 -> Data Type Conversion/1
  Memory1/1 -> MinMax1/2
  In1/1 -> ROOut1/1
  [out1] -> ROOut1/2
  MinMax/1 -> Out1/1
  Constant2/1 -> MinMax/2
  Constant3/1 -> MinMax/3

== system c00007M_harness/Eval18 ==
  In1 : Inport
  Constant2 : Constant
  Constant3 : Constant
  Data Type Conversion : DataTypeConversion
  Memory1 : Memory  InitialCondition=1
  MinMax : MinMax  Inputs=3
  MinMax1 : MinMax  Inputs=2
  ROOut1 : RelationalOperator  Operator===  OutDataTypeStr=boolean  RndMeth=Simplest
  Out1 : Outport
  wires:
  Data Type Conversion/1 -> MinMax1/1
  MinMax1/1 -> Memory1/1, MinMax/1
  ROOut1/1 -> Data Type Conversion/1
  Memory1/1 -> MinMax1/2
  In1/1 -> ROOut1/1
  [out1] -> ROOut1/2
  MinMax/1 -> Out1/1
  Constant2/1 -> MinMax/2
  Constant3/1 -> MinMax/3

== system c00007M_harness/Eval19 ==
  In1 : Inport
  Constant2 : Constant
  Constant3 : Constant
  Data Type Conversion : DataTypeConversion
  Memory1 : Memory  InitialCondition=1
  MinMax : MinMax  Inputs=3
  MinMax1 : MinMax  Inputs=2
  ROOut1 : RelationalOperator  Operator===  OutDataTypeStr=boolean  RndMeth=Simplest
  Out1 : Outport
  wires:
  Data Type Conversion/1 -> MinMax1/1
  MinMax1/1 -> Memory1/1, MinMax/1
  ROOut1/1 -> Data Type Conversion/1
  Memory1/1 -> MinMax1/2
  In1/1 -> ROOut1/1
  [out1] -> ROOut1/2
  MinMax/1 -> Out1/1
  Constant2/1 -> MinMax/2
  Constant3/1 -> MinMax/3

== system c00007M_harness/Eval2 ==
  In1 : Inport
  Constant2 : Constant
  Constant3 : Constant
  Data Type Conversion : DataTypeConversion
  Memory1 : Memory  InitialCondition=1
  MinMax : MinMax  Inputs=3
  MinMax1 : MinMax  Inputs=2
  ROOut1 : RelationalOperator  Operator===  OutDataTypeStr=boolean  RndMeth=Simplest
  Out1 : Outport
  wires:
  Data Type Conversion/1 -> MinMax1/1
  MinMax1/1 -> Memory1/1, MinMax/1
  ROOut1/1 -> Data Type Conversion/1
  Memory1/1 -> MinMax1/2
  In1/1 -> ROOut1/1
  [out1] -> ROOut1/2
  MinMax/1 -> Out1/1
  Constant2/1 -> MinMax/2
  Constant3/1 -> MinMax/3

== system c00007M_harness/Eval20 ==
  In1 : Inport
  Constant2 : Constant
  Constant3 : Constant
  Data Type Conversion : DataTypeConversion
  Memory1 : Memory  InitialCondition=1
  MinMax : MinMax  Inputs=3
  MinMax1 : MinMax  Inputs=2
  ROOut1 : RelationalOperator  Operator===  OutDataTypeStr=boolean  RndMeth=Simplest
  Out1 : Outport
  wires:
  Data Type Conversion/1 -> MinMax1/1
  MinMax1/1 -> Memory1/1, MinMax/1
  ROOut1/1 -> Data Type Conversion/1
  Memory1/1 -> MinMax1/2
  In1/1 -> ROOut1/1
  [out1] -> ROOut1/2
  MinMax/1 -> Out1/1
  Constant2/1 -> MinMax/2
  Constant3/1 -> MinMax/3

== system c00007M_harness/Eval21 ==
  In1 : Inport
  Constant2 : Constant
  Constant3 : Constant
  Data Type Conversion : DataTypeConversion
  Memory1 : Memory  InitialCondition=1
  MinMax : MinMax  Inputs=3
  MinMax1 : MinMax  Inputs=2
  ROOut1 : RelationalOperator  Operator===  OutDataTypeStr=boolean  RndMeth=Simplest
  Out1 : Outport
  wires:
  Data Type Conversion/1 -> MinMax1/1
  MinMax1/1 -> Memory1/1, MinMax/1
  ROOut1/1 -> Data Type Conversion/1
  Memory1/1 -> MinMax1/2
  In1/1 -> ROOut1/1
  [out1] -> ROOut1/2
  MinMax/1 -> Out1/1
  Constant2/1 -> MinMax/2
  Constant3/1 -> MinMax/3

== system c00007M_harness/Eval22 ==
  In1 : Inport
  Constant2 : Constant
  Constant3 : Constant
  Data Type Conversion : DataTypeConversion
  Memory1 : Memory  InitialCondition=1
  MinMax : MinMax  Inputs=3
  MinMax1 : MinMax  Inputs=2
  ROOut1 : RelationalOperator  Operator===  OutDataTypeStr=boolean  RndMeth=Simplest
  Out1 : Outport
  wires:
  Data Type Conversion/1 -> MinMax1/1
  MinMax1/1 -> Memory1/1, MinMax/1
  ROOut1/1 -> Data Type Conversion/1
  Memory1/1 -> MinMax1/2
  In1/1 -> ROOut1/1
  [out1] -> ROOut1/2
  MinMax/1 -> Out1/1
  Constant2/1 -> MinMax/2
  Constant3/1 -> MinMax/3

== system c00007M_harness/Eval23 ==
  In1 : Inport
  Constant2 : Constant
  Constant3 : Constant
  Data Type Conversion : DataTypeConversion
  Memory1 : Memory  InitialCondition=1
  MinMax : MinMax  Inputs=3
  MinMax1 : MinMax  Inputs=2
  ROOut1 : RelationalOperator  Operator===  OutDataTypeStr=boolean  RndMeth=Simplest
  Out1 : Outport
  wires:
  Data Type Conversion/1 -> MinMax1/1
  MinMax1/1 -> Memory1/1, MinMax/1
  ROOut1/1 -> Data Type Conversion/1
  Memory1/1 -> MinMax1/2
  In1/1 -> ROOut1/1
  [out1] -> ROOut1/2
  MinMax/1 -> Out1/1
  Constant2/1 -> MinMax/2
  Constant3/1 -> MinMax/3

== system c00007M_harness/Eval24 ==
  In1 : Inport
  Constant2 : Constant
  Constant3 : Constant
  Data Type Conversion : DataTypeConversion
  Memory1 : Memory  InitialCondition=1
  MinMax : MinMax  Inputs=3
  MinMax1 : MinMax  Inputs=2
  ROOut1 : RelationalOperator  Operator===  OutDataTypeStr=boolean  RndMeth=Simplest
  Out1 : Outport
  wires:
  Data Type Conversion/1 -> MinMax1/1
  MinMax1/1 -> Memory1/1, MinMax/1
  ROOut1/1 -> Data Type Conversion/1
  Memory1/1 -> MinMax1/2
  In1/1 -> ROOut1/1
  [out1] -> ROOut1/2
  MinMax/1 -> Out1/1
  Constant2/1 -> MinMax/2
  Constant3/1 -> MinMax/3

== system c00007M_harness/Eval25 ==
  In1 : Inport
  Constant2 : Constant
  Constant3 : Constant
  Data Type Conversion : DataTypeConversion
  Memory1 : Memory  InitialCondition=1
  MinMax : MinMax  Inputs=3
  MinMax1 : MinMax  Inputs=2
  ROOut1 : RelationalOperator  Operator===  OutDataTypeStr=boolean  RndMeth=Simplest
  Out1 : Outport
  wires:
  Data Type Conversion/1 -> MinMax1/1
  MinMax1/1 -> Memory1/1, MinMax/1
  ROOut1/1 -> Data Type Conversion/1
  Memory1/1 -> MinMax1/2
  In1/1 -> ROOut1/1
  [out1] -> ROOut1/2
  MinMax/1 -> Out1/1
  Constant2/1 -> MinMax/2
  Constant3/1 -> MinMax/3

== system c00007M_harness/Eval26 ==
  In1 : Inport
  Constant2 : Constant
  Constant3 : Constant
  Data Type Conversion : DataTypeConversion
  Memory1 : Memory  InitialCondition=1
  MinMax : MinMax  Inputs=3
  MinMax1 : MinMax  Inputs=2
  ROOut1 : RelationalOperator  Operator===  OutDataTypeStr=boolean  RndMeth=Simplest
  Out1 : Outport
  wires:
  Data Type Conversion/1 -> MinMax1/1
  MinMax1/1 -> Memory1/1, MinMax/1
  ROOut1/1 -> Data Type Conversion/1
  Memory1/1 -> MinMax1/2
  In1/1 -> ROOut1/1
  [out1] -> ROOut1/2
  MinMax/1 -> Out1/1
  Constant2/1 -> MinMax/2
  Constant3/1 -> MinMax/3

== system c00007M_harness/Eval27 ==
  In1 : Inport
  Constant2 : Constant
  Constant3 : Constant
  Data Type Conversion : DataTypeConversion
  Memory1 : Memory  InitialCondition=1
  MinMax : MinMax  Inputs=3
  MinMax1 : MinMax  Inputs=2
  ROOut1 : RelationalOperator  Operator===  OutDataTypeStr=boolean  RndMeth=Simplest
  Out1 : Outport
  wires:
  Data Type Conversion/1 -> MinMax1/1
  MinMax1/1 -> Memory1/1, MinMax/1
  ROOut1/1 -> Data Type Conversion/1
  Memory1/1 -> MinMax1/2
  In1/1 -> ROOut1/1
  [out1] -> ROOut1/2
  MinMax/1 -> Out1/1
  Constant2/1 -> MinMax/2
  Constant3/1 -> MinMax/3

== system c00007M_harness/Eval28 ==
  In1 : Inport
  Constant2 : Constant
  Constant3 : Constant
  Data Type Conversion : DataTypeConversion
  Memory1 : Memory  InitialCondition=1
  MinMax : MinMax  Inputs=3
  MinMax1 : MinMax  Inputs=2
  ROOut1 : RelationalOperator  Operator===  OutDataTypeStr=boolean  RndMeth=Simplest
  Out1 : Outport
  wires:
  Data Type Conversion/1 -> MinMax1/1
  MinMax1/1 -> Memory1/1, MinMax/1
  ROOut1/1 -> Data Type Conversion/1
  Memory1/1 -> MinMax1/2
  In1/1 -> ROOut1/1
  [out1] -> ROOut1/2
  MinMax/1 -> Out1/1
  Constant2/1 -> MinMax/2
  Constant3/1 -> MinMax/3

== system c00007M_harness/Eval29 ==
  In1 : Inport
  Constant2 : Constant
  Constant3 : Constant
  Data Type Conversion : DataTypeConversion
  Memory1 : Memory  InitialCondition=1
  MinMax : MinMax  Inputs=3
  MinMax1 : MinMax  Inputs=2
  ROOut1 : RelationalOperator  Operator===  OutDataTypeStr=boolean  RndMeth=Simplest
  Out1 : Outport
  wires:
  Data Type Conversion/1 -> MinMax1/1
  MinMax1/1 -> Memory1/1, MinMax/1
  ROOut1/1 -> Data Type Conversion/1
  Memory1/1 -> MinMax1/2
  In1/1 -> ROOut1/1
  [out1] -> ROOut1/2
  MinMax/1 -> Out1/1
  Constant2/1 -> MinMax/2
  Constant3/1 -> MinMax/3

== system c00007M_harness/Eval3 ==
  In1 : Inport
  Constant2 : Constant
  Constant3 : Constant
  Data Type Conversion : DataTypeConversion
  Memory1 : Memory  InitialCondition=1
  MinMax : MinMax  Inputs=3
  MinMax1 : MinMax  Inputs=2
  ROOut1 : RelationalOperator  Operator===  OutDataTypeStr=boolean  RndMeth=Simplest
  Out1 : Outport
  wires:
  Data Type Conversion/1 -> MinMax1/1
  MinMax1/1 -> Memory1/1, MinMax/1
  ROOut1/1 -> Data Type Conversion/1
  Memory1/1 -> MinMax1/2
  In1/1 -> ROOut1/1
  [out1] -> ROOut1/2
  MinMax/1 -> Out1/1
  Constant2/1 -> MinMax/2
  Constant3/1 -> MinMax/3

== system c00007M_harness/Eval30 ==
  In1 : Inport
  Constant2 : Constant
  Constant3 : Constant
  Data Type Conversion : DataTypeConversion
  Memory1 : Memory  InitialCondition=1
  MinMax : MinMax  Inputs=3
  MinMax1 : MinMax  Inputs=2
  ROOut1 : RelationalOperator  Operator===  OutDataTypeStr=boolean  RndMeth=Simplest
  Out1 : Outport
  wires:
  Data Type Conversion/1 -> MinMax1/1
  MinMax1/1 -> Memory1/1, MinMax/1
  ROOut1/1 -> Data Type Conversion/1
  Memory1/1 -> MinMax1/2
  In1/1 -> ROOut1/1
  [out1] -> ROOut1/2
  MinMax/1 -> Out1/1
  Constant2/1 -> MinMax/2
  Constant3/1 -> MinMax/3

== system c00007M_harness/Eval31 ==
  In1 : Inport
  Constant2 : Constant
  Constant3 : Constant
  Data Type Conversion : DataTypeConversion
  Memory1 : Memory  InitialCondition=1
  MinMax : MinMax  Inputs=3
  MinMax1 : MinMax  Inputs=2
  ROOut1 : RelationalOperator  Operator===  OutDataTypeStr=boolean  RndMeth=Simplest
  Out1 : Outport
  wires:
  Data Type Conversion/1 -> MinMax1/1
  MinMax1/1 -> Memory1/1, MinMax/1
  ROOut1/1 -> Data Type Conversion/1
  Memory1/1 -> MinMax1/2
  In1/1 -> ROOut1/1
  [out1] -> ROOut1/2
  MinMax/1 -> Out1/1
  Constant2/1 -> MinMax/2
  Constant3/1 -> MinMax/3

== system c00007M_harness/Eval32 ==
  In1 : Inport
  Constant2 : Constant
  Constant3 : Constant
  Data Type Conversion : DataTypeConversion
  Memory1 : Memory  InitialCondition=1
  MinMax : MinMax  Inputs=3
  MinMax1 : MinMax  Inputs=2
  ROOut1 : RelationalOperator  Operator===  OutDataTypeStr=boolean  RndMeth=Simplest
  Out1 : Outport
  wires:
  Data Type Conversion/1 -> MinMax1/1
  MinMax1/1 -> Memory1/1, MinMax/1
  ROOut1/1 -> Data Type Conversion/1
  Memory1/1 -> MinMax1/2
  In1/1 -> ROOut1/1
  [out1] -> ROOut1/2
  MinMax/1 -> Out1/1
  Constant2/1 -> MinMax/2
  Constant3/1 -> MinMax/3

== system c00007M_harness/Eval33 ==
  In1 : Inport
  Constant2 : Constant
  Constant3 : Constant
  Data Type Conversion : DataTypeConversion
  Memory1 : Memory  InitialCondition=1
  MinMax : MinMax  Inputs=3
  MinMax1 : MinMax  Inputs=2
  ROOut1 : RelationalOperator  Operator===  OutDataTypeStr=boolean  RndMeth=Simplest
  Out1 : Outport
  wires:
  Data Type Conversion/1 -> MinMax1/1
  MinMax1/1 -> Memory1/1, MinMax/1
  ROOut1/1 -> Data Type Conversion/1
  Memory1/1 -> MinMax1/2
  In1/1 -> ROOut1/1
  [out1] -> ROOut1/2
  MinMax/1 -> Out1/1
  Constant2/1 -> MinMax/2
  Constant3/1 -> MinMax/3

== system c00007M_harness/Eval34 ==
  In1 : Inport
  Constant2 : Constant
  Constant3 : Constant
  Data Type Conversion : DataTypeConversion
  Memory1 : Memory  InitialCondition=1
  MinMax : MinMax  Inputs=3
  MinMax1 : MinMax  Inputs=2
  ROOut1 : RelationalOperator  Operator===  OutDataTypeStr=boolean  RndMeth=Simplest
  Out1 : Outport
  wires:
  Data Type Conversion/1 -> MinMax1/1
  MinMax1/1 -> Memory1/1, MinMax/1
  ROOut1/1 -> Data Type Conversion/1
  Memory1/1 -> MinMax1/2
  In1/1 -> ROOut1/1
  [out1] -> ROOut1/2
  MinMax/1 -> Out1/1
  Constant2/1 -> MinMax/2
  Constant3/1 -> MinMax/3

== system c00007M_harness/Eval35 ==
  In1 : Inport
  Constant2 : Constant
  Constant3 : Constant
  Data Type Conversion : DataTypeConversion
  Memory1 : Memory  InitialCondition=1
  MinMax : MinMax  Inputs=3
  MinMax1 : MinMax  Inputs=2
  ROOut1 : RelationalOperator  Operator===  OutDataTypeStr=boolean  RndMeth=Simplest
  Out1 : Outport
  wires:
  Data Type Conversion/1 -> MinMax1/1
  MinMax1/1 -> Memory1/1, MinMax/1
  ROOut1/1 -> Data Type Conversion/1
  Memory1/1 -> MinMax1/2
  In1/1 -> ROOut1/1
  [out1] -> ROOut1/2
  MinMax/1 -> Out1/1
  Constant2/1 -> MinMax/2
  Constant3/1 -> MinMax/3

== system c00007M_harness/Eval36 ==
  In1 : Inport
  Constant2 : Constant
  Constant3 : Constant
  Data Type Conversion : DataTypeConversion
  Memory1 : Memory  InitialCondition=1
  MinMax : MinMax  Inputs=3
  MinMax1 : MinMax  Inputs=2
  ROOut1 : RelationalOperator  Operator===  OutDataTypeStr=boolean  RndMeth=Simplest
  Out1 : Outport
  wires:
  Data Type Conversion/1 -> MinMax1/1
  MinMax1/1 -> Memory1/1, MinMax/1
  ROOut1/1 -> Data Type Conversion/1
  Memory1/1 -> MinMax1/2
  In1/1 -> ROOut1/1
  [out1] -> ROOut1/2
  MinMax/1 -> Out1/1
  Constant2/1 -> MinMax/2
  Constant3/1 -> MinMax/3

== system c00007M_harness/Eval37 ==
  In1 : Inport
  Constant2 : Constant
  Constant3 : Constant
  Data Type Conversion : DataTypeConversion
  Memory1 : Memory  InitialCondition=1
  MinMax : MinMax  Inputs=3
  MinMax1 : MinMax  Inputs=2
  ROOut1 : RelationalOperator  Operator===  OutDataTypeStr=boolean  RndMeth=Simplest
  Out1 : Outport
  wires:
  Data Type Conversion/1 -> MinMax1/1
  MinMax1/1 -> Memory1/1, MinMax/1
  ROOut1/1 -> Data Type Conversion/1
  Memory1/1 -> MinMax1/2
  In1/1 -> ROOut1/1
  [out1] -> ROOut1/2
  MinMax/1 -> Out1/1
  Constant2/1 -> MinMax/2
  Constant3/1 -> MinMax/3

== system c00007M_harness/Eval38 ==
  In1 : Inport
  Constant2 : Constant
  Constant3 : Constant
  Data Type Conversion : DataTypeConversion
  Memory1 : Memory  InitialCondition=1
  MinMax : MinMax  Inputs=3
  MinMax1 : MinMax  Inputs=2
  ROOut1 : RelationalOperator  Operator===  OutDataTypeStr=boolean  RndMeth=Simplest
  Out1 : Outport
  wires:
  Data Type Conversion/1 -> MinMax1/1
  MinMax1/1 -> Memory1/1, MinMax/1
  ROOut1/1 -> Data Type Conversion/1
  Memory1/1 -> MinMax1/2
  In1/1 -> ROOut1/1
  [out1] -> ROOut1/2
  MinMax/1 -> Out1/1
  Constant2/1 -> MinMax/2
  Constant3/1 -> MinMax/3

== system c00007M_harness/Eval39 ==
  In1 : Inport
  Constant2 : Constant
  Constant3 : Constant
  Data Type Conversion : DataTypeConversion
  Memory1 : Memory  InitialCondition=1
  MinMax : MinMax  Inputs=3
  MinMax1 : MinMax  Inputs=2
  ROOut1 : RelationalOperator  Operator===  OutDataTypeStr=boolean  RndMeth=Simplest
  Out1 : Outport
  wires:
  Data Type Conversion/1 -> MinMax1/1
  MinMax1/1 -> Memory1/1, MinMax/1
  ROOut1/1 -> Data Type Conversion/1
  Memory1/1 -> MinMax1/2
  In1/1 -> ROOut1/1
  [out1] -> ROOut1/2
  MinMax/1 -> Out1/1
  Constant2/1 -> MinMax/2
  Constant3/1 -> MinMax/3

== system c00007M_harness/Eval4 ==
  In1 : Inport
  Constant2 : Constant
  Constant3 : Constant
  Data Type Conversion : DataTypeConversion
  Memory1 : Memory  InitialCondition=1
  MinMax : MinMax  Inputs=3
  MinMax1 : MinMax  Inputs=2
  ROOut1 : RelationalOperator  Operator===  OutDataTypeStr=boolean  RndMeth=Simplest
  Out1 : Outport
  wires:
  Data Type Conversion/1 -> MinMax1/1
  MinMax1/1 -> Memory1/1, MinMax/1
  ROOut1/1 -> Data Type Conversion/1
  Memory1/1 -> MinMax1/2
  In1/1 -> ROOut1/1
  [out1] -> ROOut1/2
  MinMax/1 -> Out1/1
  Constant2/1 -> MinMax/2
  Constant3/1 -> MinMax/3

== system c00007M_harness/Eval40 ==
  In1 : Inport
  Constant2 : Constant
  Constant3 : Constant
  Data Type Conversion : DataTypeConversion
  Memory1 : Memory  InitialCondition=1
  MinMax : MinMax  Inputs=3
  MinMax1 : MinMax  Inputs=2
  ROOut1 : RelationalOperator  Operator===  OutDataTypeStr=boolean  RndMeth=Simplest
  Out1 : Outport
  wires:
  Data Type Conversion/1 -> MinMax1/1
  MinMax1/1 -> Memory1/1, MinMax/1
  ROOut1/1 -> Data Type Conversion/1
  Memory1/1 -> MinMax1/2
  In1/1 -> ROOut1/1
  [out1] -> ROOut1/2
  MinMax/1 -> Out1/1
  Constant2/1 -> MinMax/2
  Constant3/1 -> MinMax/3

== system c00007M_harness/Eval41 ==
  In1 : Inport
  Constant2 : Constant
  Constant3 : Constant
  Data Type Conversion : DataTypeConversion
  Memory1 : Memory  InitialCondition=1
  MinMax : MinMax  Inputs=3
  MinMax1 : MinMax  Inputs=2
  ROOut1 : RelationalOperator  Operator===  OutDataTypeStr=boolean  RndMeth=Simplest
  Out1 : Outport
  wires:
  Data Type Conversion/1 -> MinMax1/1
  MinMax1/1 -> Memory1/1, MinMax/1
  ROOut1/1 -> Data Type Conversion/1
  Memory1/1 -> MinMax1/2
  In1/1 -> ROOut1/1
  [out1] -> ROOut1/2
  MinMax/1 -> Out1/1
  Constant2/1 -> MinMax/2
  Constant3/1 -> MinMax/3

== system c00007M_harness/Eval42 ==
  In1 : Inport
  Constant2 : Constant
  Constant3 : Constant
  Data Type Conversion : DataTypeConversion
  Memory1 : Memory  InitialCondition=1
  MinMax : MinMax  Inputs=3
  MinMax1 : MinMax  Inputs=2
  ROOut1 : RelationalOperator  Operator===  OutDataTypeStr=boolean  RndMeth=Simplest
  Out1 : Outport
  wires:
  Data Type Conversion/1 -> MinMax1/1
  MinMax1/1 -> Memory1/1, MinMax/1
  ROOut1/1 -> Data Type Conversion/1
  Memory1/1 -> MinMax1/2
  In1/1 -> ROOut1/1
  [out1] -> ROOut1/2
  MinMax/1 -> Out1/1
  Constant2/1 -> MinMax/2
  Constant3/1 -> MinMax/3

== system c00007M_harness/Eval43 ==
  In1 : Inport
  Constant2 : Constant
  Constant3 : Constant
  Data Type Conversion : DataTypeConversion
  Memory1 : Memory  InitialCondition=1
  MinMax : MinMax  Inputs=3
  MinMax1 : MinMax  Inputs=2
  ROOut1 : RelationalOperator  Operator===  OutDataTypeStr=boolean  RndMeth=Simplest
  Out1 : Outport
  wires:
  Data Type Conversion/1 -> MinMax1/1
  MinMax1/1 -> Memory1/1, MinMax/1
  ROOut1/1 -> Data Type Conversion/1
  Memory1/1 -> MinMax1/2
  In1/1 -> ROOut1/1
  [out1] -> ROOut1/2
  MinMax/1 -> Out1/1
  Constant2/1 -> MinMax/2
  Constant3/1 -> MinMax/3
